simulink model "hardware_model"  (R2023a)
settings: Solver=FixedStepAuto  StartTime=0.0  StopTime=inf  FixedStep=1/50  RelTol=1e-3  EnableMultiTasking=on
undefined symbols (not defined in the file): data, id, timestamp
libraries: px4uORBlib x5
settings Model: ExtModeTrigDuration=10  Creator=The MathWorks, Inc.  LastModifiedBy=thesa
settings SolverCC: PositivePriorityOrder=on  MaxZcPerStep=1
settings OptimizationCC: EnhancedBackFolding=on  StrengthReduction=on  BooleansAsBitfields=on  PassReuseOutputArgsAs=Individual arguments  StateBitsets=on  DataBitsets=on  ZeroExternalMemoryAtStartup=off  ZeroInternalMemoryAtStartup=off  MaxStackSize=64  OptimizeBlockOrder=speed  DifferentSizesBufferReuse=on  OptimizationPriority=RAM  EfficientTunableParamExpr=on
settings DebuggingCC: ParameterTunabilityLossMsg=error
settings HardwareCC: ProdBitPerPointer=32  ProdBitPerSizeT=32  ProdBitPerPtrDiffT=32  ProdLargestAtomicInteger=Long  ProdLargestAtomicFloat=Double  ProdWordSize=32  ProdLongLongMode=on  ProdHWDeviceType=ARM Compatible->ARM Cortex
settings ModelReferenceCC: EnableRefExpFcnMdlSchedulingChecks=on  ParallelModelReferenceMATLABWorkerInit=Copy Base Workspace
settings SFSimCC: MATLABDynamicMemAlloc=off  SimTargetLang=C++
settings RTWCC: Description=Embedded Coder  SystemTargetFile=ert.tlc  HardwareBoard=PX4 Cube Orange  TLCOptions="-aInlineSetEventsForThisBaseRateFcn=TLC_FALSE -aSuppressMultiTaskScheduler=TLC_FALSE  -aRateBasedStepFcn=0"  TemplateMakefile=ert_default_tmf  Toolchain=GNU Tools for PX4 Autopilots  TargetLang=C++  DLArmComputeVersion=19.05
settings CodeAppCC: ForceParamTrailComments=on  IgnoreCustomStorageClasses=off  MaxIdLength=63  OperatorAnnotations=on  SimulinkDataObjDesc=on  SFDataObjDesc=on  InsertBlockDesc=on
settings ERTTargetCC: ExtModeTransport=3  ExtModeStaticAlloc=on  ExtModeStaticAllocSize=1024  ExtModeMexFile=ext_xcp  ExtModeIntrfLevel=Level2 - Open

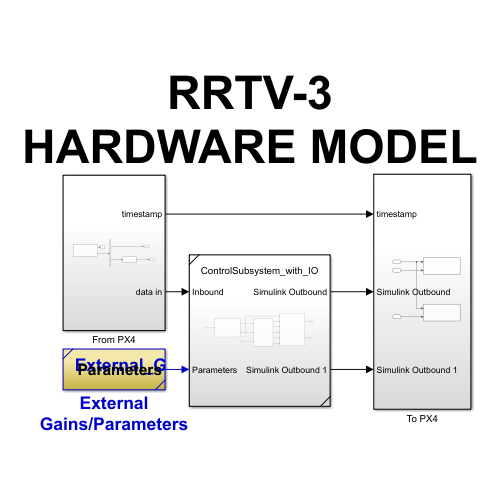
[thumbnail: Simulink's stored preview of the top-level diagram]
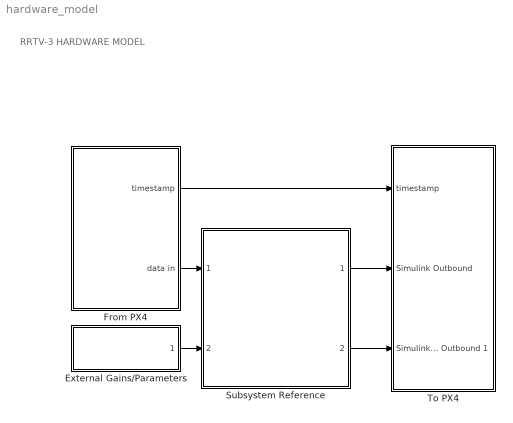
== system hardware_model ==
  note: RRTV-3
      | HARDWARE MODEL
  External Gains/Parameters : Subsystem  ReferencedSubsystem=External_Gains_Parameters
  From PX4 : Subsystem
  Subsystem Reference : Subsystem  ReferencedSubsystem=ControlSubsystem_with_IO
  To PX4 : Subsystem
  wires:
  From PX4/2(data in) -> Subsystem Reference/1
  Subsystem Reference/1 -> To PX4/2(Simulink Outbound)
  External Gains/Parameters/1 -> Subsystem Reference/2
  Subsystem Reference/2 -> To PX4/3(Simulink Outbound 1)
  From PX4/1(timestamp) -> To PX4/1(timestamp)

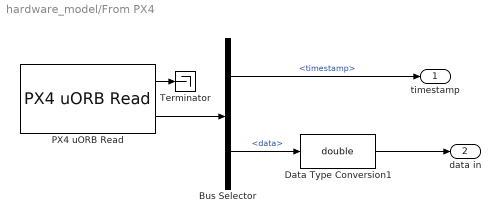
== system hardware_model/From PX4 ==
  Bus Selector : BusSelector  OutputSignals=timestamp,data
  Data Type Conversion1 : DataTypeConversion  OutDataTypeStr=double  SaturateOnIntegerOverflow=off  RndMeth=Floor
  PX4 uORB Read : px4uORBlib/PX4 uORB Read  uORBTopic=debug_array  selectInstance=simulink_inbound  SampleTime=-1  BlockingMode=off  BlockTimeout=1e-3
  Terminator : Terminator
  timestamp : Outport
  data in : Outport  Port=2
  wires:
  PX4 uORB Read/1 -> Terminator/1
  PX4 uORB Read/2 -> Bus Selector/1
  Bus Selector/2 -> Data Type Conversion1/1  "<data>"
  Data Type Conversion1/1 -> data in/1
  Bus Selector/1 -> timestamp/1  "<timestamp>"

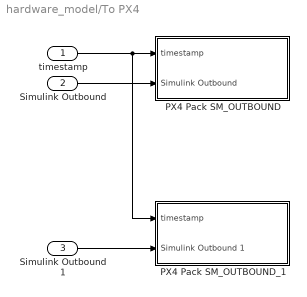
== system hardware_model/To PX4 ==
  timestamp : Inport
  Simulink Outbound : Inport  Port=2
  Simulink Outbound 1 : Inport  Port=3
  PX4 Pack SM_OUTBOUND : Subsystem
  PX4 Pack SM_OUTBOUND_1 : Subsystem
  wires:
  Simulink Outbound/1 -> PX4 Pack SM_OUTBOUND/2(Simulink Outbound)
  Simulink Outbound 1/1 -> PX4 Pack SM_OUTBOUND_1/2(Simulink Outbound 1)
  timestamp/1 -> PX4 Pack SM_OUTBOUND_1/1(timestamp), PX4 Pack SM_OUTBOUND/1(timestamp)

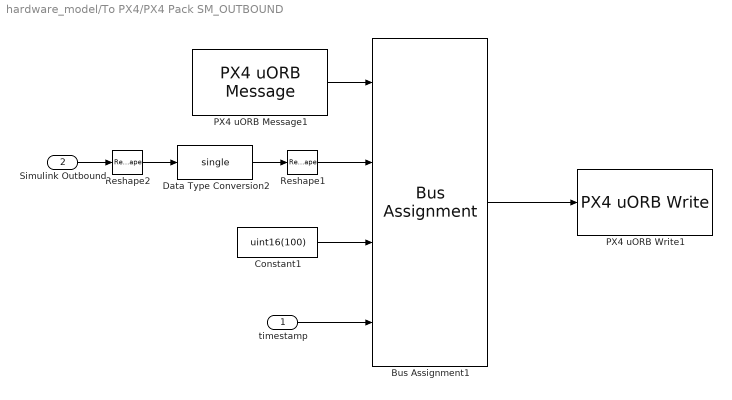
== system hardware_model/To PX4/PX4 Pack SM_OUTBOUND ==
  timestamp : Inport
  Simulink Outbound : Inport  Port=2
  Bus Assignment1 : BusAssignment  AssignedSignals=data,id,timestamp
  Constant1 : Constant  Value=uint16(100)  OutDataTypeStr=uint16
  Data Type Conversion2 : DataTypeConversion  OutDataTypeStr=single  SaturateOnIntegerOverflow=off  RndMeth=Floor
  PX4 uORB Message1 : px4uORBlib/PX4 uORB Message  uORBTopic=debug_array  SampleTime=inf  selectInstance=vehicle_gps_position
  PX4 uORB Write1 : px4uORBlib/PX4 uORB Write  uORBTopic=debug_array  selectInstance=simulink_outbound  MessageQueueLen=1
  Reshape1 : Reshape
  Reshape2 : Reshape
  wires:
  Data Type Conversion2/1 -> Reshape1/1
  Constant1/1 -> Bus Assignment1/3
  Reshape2/1 -> Data Type Conversion2/1
  Bus Assignment1/1 -> PX4 uORB Write1/1
  PX4 uORB Message1/1 -> Bus Assignment1/1
  Reshape1/1 -> Bus Assignment1/2
  Simulink Outbound/1 -> Reshape2/1
  timestamp/1 -> Bus Assignment1/4

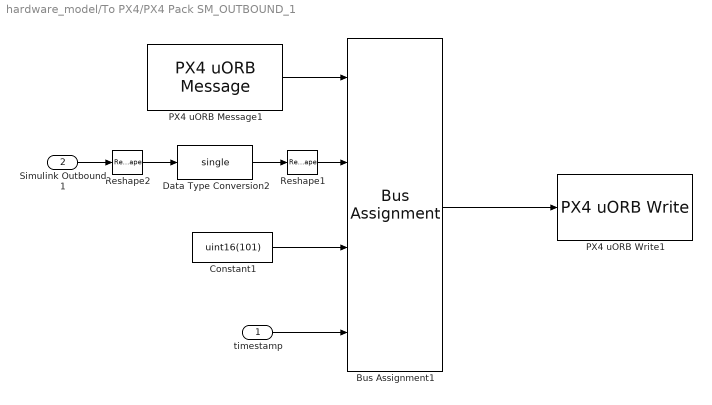
== system hardware_model/To PX4/PX4 Pack SM_OUTBOUND_1 ==
  timestamp : Inport
  Simulink Outbound 1 : Inport  Port=2
  Bus Assignment1 : BusAssignment  AssignedSignals=data,id,timestamp
  Constant1 : Constant  Value=uint16(101)  OutDataTypeStr=uint16
  Data Type Conversion2 : DataTypeConversion  OutDataTypeStr=single  SaturateOnIntegerOverflow=off  RndMeth=Floor
  PX4 uORB Message1 : px4uORBlib/PX4 uORB Message  uORBTopic=debug_array  SampleTime=inf  selectInstance=vehicle_gps_position
  PX4 uORB Write1 : px4uORBlib/PX4 uORB Write  uORBTopic=debug_array  selectInstance=simulink_outbound_1  MessageQueueLen=1
  Reshape1 : Reshape
  Reshape2 : Reshape
  wires:
  Simulink Outbound 1/1 -> Reshape2/1
  Reshape1/1 -> Bus Assignment1/2
  PX4 uORB Message1/1 -> Bus Assignment1/1
  Bus Assignment1/1 -> PX4 uORB Write1/1
  Reshape2/1 -> Data Type Conversion2/1
  Constant1/1 -> Bus Assignment1/3
  Data Type Conversion2/1 -> Reshape1/1
  timestamp/1 -> Bus Assignment1/4
